simulink model "ARDroneHover"  (R2013b)
settings: Solver=ode1  StartTime=0.0  StopTime=inf  FixedStep=sampleTime  RelTol=1e-3
values from neighbouring files (symbols this model uses):
  sampleTime = 0.065    [setupHover.m]    (also in setupWPTracking.m)
libraries: ARBlocks x3
CloseFcn:
  | rtwprivate ssgencode ModelCloseRequest Good_NL_model
settings Model: SimulationMode=external  ExtModeTrigDuration=100000  Creator=Paul  LastModifiedBy=david
settings DataIOCC: SignalLoggingSaveFormat=ModelDataLogs  TimeSaveName=time
settings OptimizationCC: ExpressionDepthLimit=2147483647  InitFltsAndDblsToZero=on
settings DebuggingCC: FcnCallInpInsideContextMsg=UseLocalSettings  StateNameClashWarn=warning
settings HardwareCC: ProdIntDivRoundTo=Zero  ProdEndianess=LittleEndian  ProdHWDeviceType=Generic->32-bit x86 compatible
settings RTWCC: SystemTargetFile=rtwin.tlc  TemplateMakefile=rtwin.tmf  Description=Real-Time Windows Target  ProcessScript=rtwin_make_rtw_hook  RTWCompilerOptimization=On
settings CodeAppCC: MaxIdLength=95
settings RTWinTargetCC: TargetLibSuffix=_rtwin.lib  TargetPreCompLibLocation=C:\Program Files\MATLAB\R2013b2\toolbox\rtw\targets\rtwin\lib\win64  CodeReplacementLibrary=ANSI_C  RTWinDir=C:/PROGRA~1/MATLAB/R2013b2/toolbox/rtw/targets/rtwin  TargetArch=win64

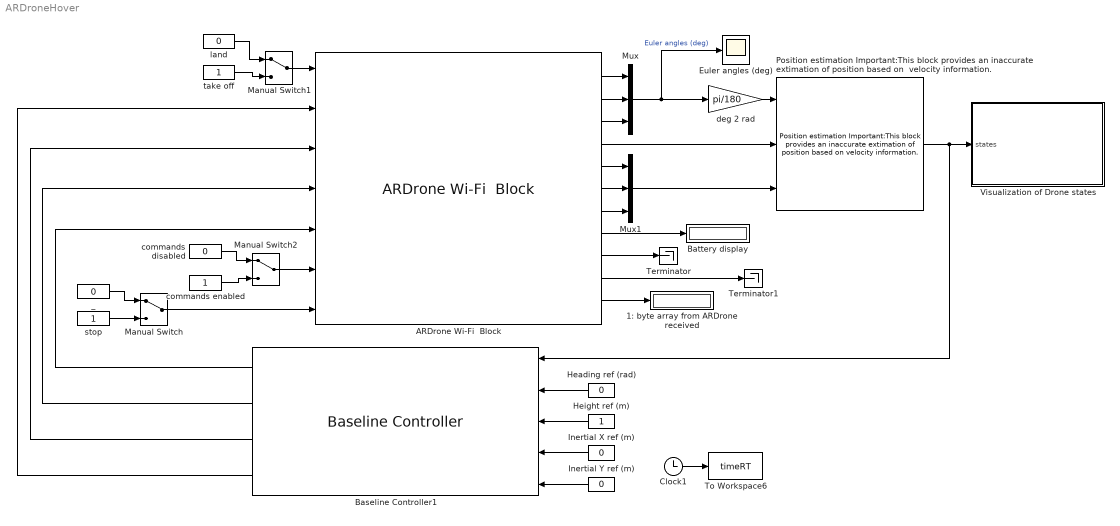
== system ARDroneHover ==
  "1: byte array from ARDrone received " : Display
  ARDrone Wi-Fi  Block : ARBlocks/ARDrone Wi-Fi  Block
  Baseline Controller1 : ARBlocks/Baseline Controller
  Battery display : Display
  Clock1 : Clock
  Euler angles (deg) : Scope
      settings: YMin=-10  YMax=120  MaxDataPoints=500000
  Heading ref (rad) : Constant  Value=0
  Height ref (m) : Constant
  Inertial X ref (m) : Constant  Value=0
  Inertial Y ref (m) : Constant  Value=0
  Manual Switch : ManualSwitch
  Manual Switch1 : ManualSwitch
  Manual Switch2 : ManualSwitch
  Mux : Mux  Inputs=3
  Mux1 : Mux  Inputs=3
  "Position estimation Important:This block provides an inaccurate extimation of position based on  velocity information. " : ARBlocks/Position estimation Important:This block provides an  inaccurate extimation of position  based on  velocity information. 
  Terminator : Terminator
  Terminator1 : Terminator
  To Workspace6 : ToWorkspace  VariableName=timeRT  SampleTime=sampleTime
  Visualization of Drone states : Subsystem
  _ : Constant  Value=0
  commands disabled : Constant  Value=0
  commands enabled : Constant
  deg 2 rad : Gain  Gain=pi/180
  land : Constant  Value=0
  stop : Constant
  take off : Constant
  wires:
  _/1 -> Manual Switch/1
  stop/1 -> Manual Switch/2
  land/1 -> Manual Switch1/1
  take off/1 -> Manual Switch1/2
  commands disabled/1 -> Manual Switch2/1
  commands enabled/1 -> Manual Switch2/2
  Manual Switch1/1 -> ARDrone Wi-Fi  Block/1
  Manual Switch2/1 -> ARDrone Wi-Fi  Block/6
  Manual Switch/1 -> ARDrone Wi-Fi  Block/7
  ARDrone Wi-Fi  Block/1 -> Mux/1
  ARDrone Wi-Fi  Block/2 -> Mux/2
  ARDrone Wi-Fi  Block/5 -> Mux1/1
  ARDrone Wi-Fi  Block/6 -> Mux1/2
  ARDrone Wi-Fi  Block/7 -> Mux1/3
  Mux/1 -> Euler angles (deg)/1, deg 2 rad/1  "Euler angles (deg)"
  ARDrone Wi-Fi  Block/8 -> Battery display/1
  Baseline Controller1/1 -> ARDrone Wi-Fi  Block/5
  Baseline Controller1/3 -> ARDrone Wi-Fi  Block/3
  "Position estimation Important:This block provides an inaccurate extimation of position based on  velocity information. "/1 -> Visualization of Drone states/1(states), Baseline Controller1/1
  deg 2 rad/1 -> "Position estimation Important:This block provides an inaccurate extimation of position based on  velocity information. "/1
  ARDrone Wi-Fi  Block/4 -> "Position estimation Important:This block provides an inaccurate extimation of position based on  velocity information. "/2
  Mux1/1 -> "Position estimation Important:This block provides an inaccurate extimation of position based on  velocity information. "/3
  Baseline Controller1/4 -> ARDrone Wi-Fi  Block/2
  ARDrone Wi-Fi  Block/3 -> Mux/3
  ARDrone Wi-Fi  Block/9 -> Terminator/1
  ARDrone Wi-Fi  Block/10 -> Terminator1/1
  ARDrone Wi-Fi  Block/11 -> "1: byte array from ARDrone received "/1
  Baseline Controller1/2 -> ARDrone Wi-Fi  Block/4
  Clock1/1 -> To Workspace6/1
  Height ref (m)/1 -> Baseline Controller1/3
  Inertial X ref (m)/1 -> Baseline Controller1/4
  Inertial Y ref (m)/1 -> Baseline Controller1/5
  Heading ref (rad)/1 -> Baseline Controller1/2

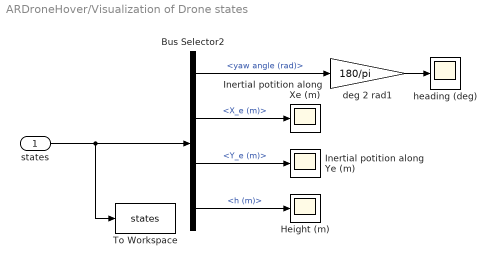
== system ARDroneHover/Visualization of Drone states ==
  states : Inport
  Bus Selector2 : BusSelector  OutputSignals=yaw angle (rad),X_e (m),Y_e (m),h (m)
  Height (m) : Scope
      settings: YMin=-22.5  YMax=22.5  SaveName=ScopeData5  MaxDataPoints=500000
  Inertial potition along Xe (m) : Scope
      settings: YMin=-22.5  YMax=22.5  SaveName=ScopeData3  MaxDataPoints=500000
  Inertial potition along Ye (m) : Scope
      settings: YMin=-22.5  YMax=22.5  SaveName=ScopeData4  MaxDataPoints=500000
  To Workspace : ToWorkspace  VariableName=states  SampleTime=-1  SaveFormat=Structure With Time
  deg 2 rad1 : Gain  Gain=180/pi
  heading (deg) : Scope
      settings: YMin=-22.5  YMax=22.5  SaveName=ScopeData2  MaxDataPoints=500000
  wires:
  states/1 -> To Workspace/1, Bus Selector2/1
  Bus Selector2/1 -> deg 2 rad1/1  "<yaw angle (rad)>"
  Bus Selector2/2 -> Inertial potition along Xe (m)/1  "<X_e (m)>"
  Bus Selector2/3 -> Inertial potition along Ye (m)/1  "<Y_e (m)>"
  Bus Selector2/4 -> Height (m)/1  "<h (m)>"
  deg 2 rad1/1 -> heading (deg)/1
